simulink model "MIMO_FIXED"  (R2017a)
settings: Solver=VariableStepAuto  StartTime=0.0  StopTime=1000  RelTol=1e-3
libraries: dspsigops x80, commchan3 x4, commdigbbndpm3 x2, commfilt2 x2, commsink2 x1, commutil2 x1
(part 2 of 6)

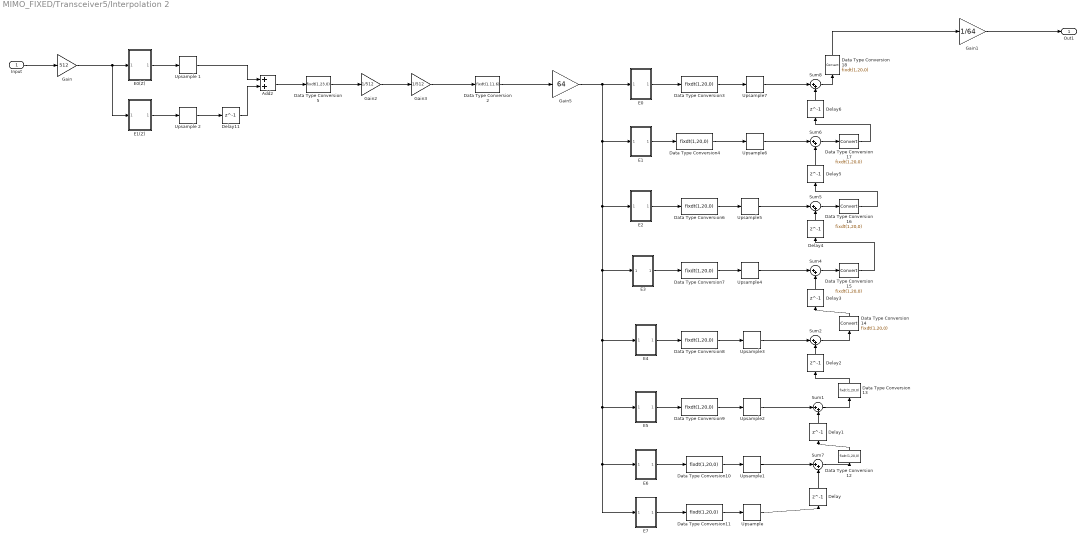
== system MIMO_FIXED/Transceiver5/Interpolation 2 ==
  Input : Inport
  Add2 : Sum
  Data Type Conversion{3..4,6..18} (15 alike) : DataTypeConversion  OutDataTypeStr=fixdt(1,20,0)  SaturateOnIntegerOverflow=on
  Data Type Conversion2 : DataTypeConversion  OutDataTypeStr=fixdt(1,11,6)  SaturateOnIntegerOverflow=on
  Data Type Conversion5 : DataTypeConversion  OutDataTypeStr=fixdt(1,23,0)  SaturateOnIntegerOverflow=on
  Delay{,1..6,11} (8 alike) : Delay  DelayLength=1
  E0 : Subsystem
  E0(Z) : Subsystem
  E1 : Subsystem
  E1(Z) : Subsystem
  E2 : Subsystem
  E3 : Subsystem
  E4 : Subsystem
  E5 : Subsystem
  E6 : Subsystem
  E7 : Subsystem
  Gain : Gain  Gain=512
  Gain1 : Gain  Gain=1/64
  Gain2 : Gain  Gain=1/512
  Gain3 : Gain  Gain=1/512
  Gain5 : Gain  Gain=64
  Sum{1..2,4..8} (7 alike) : Sum  Inputs=|++
  Upsample{,1..7} (8 alike) : dspsigops/Upsample  N=8  phase=0  RateOptions=Allow multirate processing  ic=0  mode=Unused parameter value
  Upsample 1 : dspsigops/Upsample  N=2  phase=0  RateOptions=Allow multirate processing  ic=0  mode=Unused parameter value
  Upsample 2 : dspsigops/Upsample  N=2  phase=0  RateOptions=Allow multirate processing  ic=0  mode=Unused parameter value
  Out1 : Outport
  wires:
  Upsample/1 -> Delay/1
  Delay5/1 -> Sum6/2
  Upsample6/1 -> Sum6/1
  Delay4/1 -> Sum5/2
  Delay3/1 -> Sum4/2
  Sum6/1 -> Data Type Conversion17/1
  Upsample1/1 -> Sum7/1
  Upsample2/1 -> Sum1/1
  Input/1 -> Gain/1
  Upsample 2/1 -> Delay11/1
  Delay6/1 -> Sum8/2
  E0/1(Out1) -> Data Type Conversion3/1
  Delay/1 -> Sum7/2
  E1/1(Out1) -> Data Type Conversion4/1
  Delay1/1 -> Sum1/2
  Sum5/1 -> Data Type Conversion16/1
  Sum4/1 -> Data Type Conversion15/1
  Upsample5/1 -> Sum5/1
  Upsample 1/1 -> Add2/1
  Upsample4/1 -> Sum4/1
  Delay11/1 -> Add2/2
  Sum2/1 -> Data Type Conversion14/1
  E3/1(Out1) -> Data Type Conversion7/1
  Delay2/1 -> Sum2/2
  Upsample7/1 -> Sum8/1
  Upsample3/1 -> Sum2/1
  E2/1(Out1) -> Data Type Conversion6/1
  E4/1(Out1) -> Data Type Conversion8/1
  E0(Z)/1(Out1) -> Upsample 1/1
  Data Type Conversion3/1 -> Upsample7/1
  Data Type Conversion4/1 -> Upsample6/1
  Data Type Conversion6/1 -> Upsample5/1
  Data Type Conversion7/1 -> Upsample4/1
  Data Type Conversion8/1 -> Upsample3/1
  Data Type Conversion9/1 -> Upsample2/1
  Data Type Conversion10/1 -> Upsample1/1
  Data Type Conversion11/1 -> Upsample/1
  Data Type Conversion12/1 -> Delay1/1
  Sum7/1 -> Data Type Conversion12/1
  Data Type Conversion13/1 -> Delay2/1
  Data Type Conversion14/1 -> Delay3/1
  Sum1/1 -> Data Type Conversion13/1
  Data Type Conversion15/1 -> Delay4/1
  Data Type Conversion16/1 -> Delay5/1
  Data Type Conversion17/1 -> Delay6/1
  Data Type Conversion18/1 -> Gain1/1
  Sum8/1 -> Data Type Conversion18/1
  E5/1(Out1) -> Data Type Conversion9/1
  E6/1(Out1) -> Data Type Conversion10/1
  E7/1(Out1) -> Data Type Conversion11/1
  Gain5/1 -> E0/1(In1), E7/1(In1), E6/1(In1), E5/1(In1), E4/1(In1), E3/1(In1), E2/1(In1), E1/1(In1)
  Gain1/1 -> Out1/1
  Gain/1 -> E0(Z)/1(Input), E1(Z)/1(Input1)
  Data Type Conversion2/1 -> Gain5/1
  Gain2/1 -> Gain3/1
  E1(Z)/1(Output) -> Upsample 2/1
  Gain3/1 -> Data Type Conversion2/1
  Add2/1 -> Data Type Conversion5/1
  Data Type Conversion5/1 -> Gain2/1

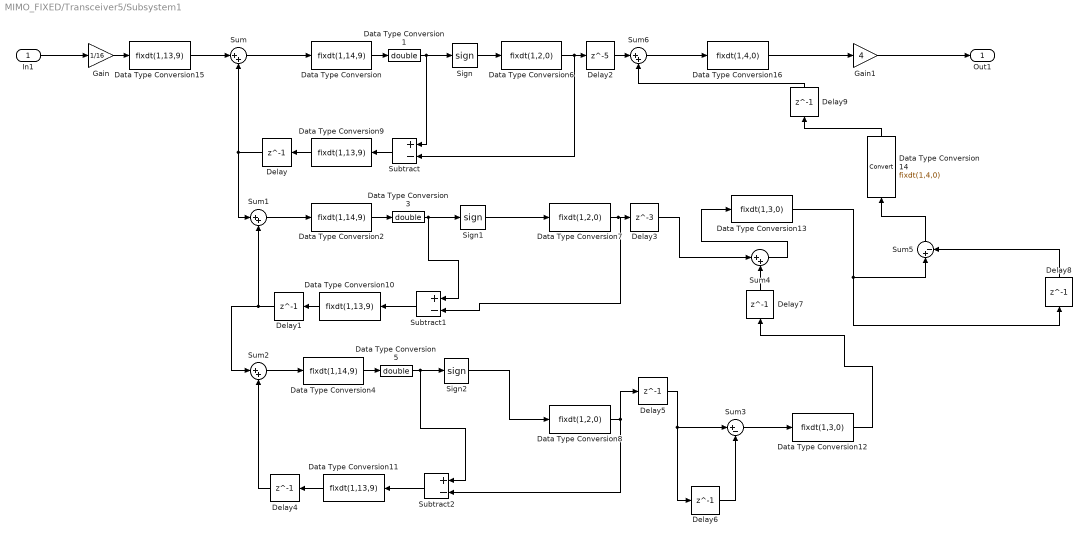
== system MIMO_FIXED/Transceiver5/Subsystem1 ==
  In1 : Inport
  Data Type Conversion : DataTypeConversion  OutDataTypeStr=fixdt(1,14,9)
  Data Type Conversion1 : DataTypeConversion  OutDataTypeStr=double
  Data Type Conversion{9..11,15} (4 alike) : DataTypeConversion  OutDataTypeStr=fixdt(1,13,9)
  Data Type Conversion12 : DataTypeConversion  OutDataTypeStr=fixdt(1,3,0)
  Data Type Conversion13 : DataTypeConversion  OutDataTypeStr=fixdt(1,3,0)
  Data Type Conversion14 : DataTypeConversion  OutDataTypeStr=fixdt(1,4,0)
  Data Type Conversion16 : DataTypeConversion  OutDataTypeStr=fixdt(1,4,0)
  Data Type Conversion2 : DataTypeConversion  OutDataTypeStr=fixdt(1,14,9)
  Data Type Conversion3 : DataTypeConversion  OutDataTypeStr=double
  Data Type Conversion4 : DataTypeConversion  OutDataTypeStr=fixdt(1,14,9)
  Data Type Conversion5 : DataTypeConversion  OutDataTypeStr=double
  Data Type Conversion6 : DataTypeConversion  OutDataTypeStr=fixdt(1,2,0)
  Data Type Conversion7 : DataTypeConversion  OutDataTypeStr=fixdt(1,2,0)
  Data Type Conversion8 : DataTypeConversion  OutDataTypeStr=fixdt(1,2,0)
  Delay{,1,4..9} (8 alike) : Delay  DelayLength=1
  Delay2 : Delay  DelayLength=5
  Delay3 : Delay  DelayLength=3
  Gain : Gain  Gain=1/16
  Gain1 : Gain  Gain=4
  Sign : Signum
  Sign1 : Signum
  Sign2 : Signum
  Subtract : Sum  Inputs=+-
  Subtract1 : Sum  Inputs=+-
  Subtract2 : Sum  Inputs=+-
  Sum{,1..2,4,6} (5 alike) : Sum  Inputs=|++
  Sum3 : Sum  Inputs=|+-
  Sum5 : Sum  Inputs=|+-
  Out1 : Outport
  wires:
  Sum/1 -> Data Type Conversion/1
  Sum2/1 -> Data Type Conversion4/1
  Delay4/1 -> Sum2/2
  Delay8/1 -> Sum5/2
  Sum4/1 -> Data Type Conversion13/1
  Subtract/1 -> Data Type Conversion9/1
  Delay5/1 -> Sum3/1, Delay6/1
  Sign1/1 -> Data Type Conversion7/1
  Delay1/1 -> Sum1/2, Sum2/1
  Sum1/1 -> Data Type Conversion2/1
  Subtract1/1 -> Data Type Conversion10/1
  Sum3/1 -> Data Type Conversion12/1
  Delay/1 -> Sum/2, Sum1/1
  Delay3/1 -> Sum4/1
  Delay7/1 -> Sum4/2
  Subtract2/1 -> Data Type Conversion11/1
  Delay6/1 -> Sum3/2
  Sum5/1 -> Data Type Conversion14/1
  Delay2/1 -> Sum6/1
  Delay9/1 -> Sum6/2
  In1/1 -> Gain/1
  Sum6/1 -> Data Type Conversion16/1
  Data Type Conversion/1 -> Data Type Conversion1/1
  Data Type Conversion1/1 -> Subtract/1, Sign/1
  Data Type Conversion2/1 -> Data Type Conversion3/1
  Data Type Conversion4/1 -> Data Type Conversion5/1
  Data Type Conversion6/1 -> Subtract/2, Delay2/1
  Data Type Conversion7/1 -> Subtract1/2, Delay3/1
  Data Type Conversion8/1 -> Delay5/1, Subtract2/2
  Data Type Conversion9/1 -> Delay/1
  Data Type Conversion10/1 -> Delay1/1
  Data Type Conversion11/1 -> Delay4/1
  Data Type Conversion12/1 -> Delay7/1
  Data Type Conversion13/1 -> Sum5/1, Delay8/1
  Data Type Conversion14/1 -> Delay9/1
  Gain/1 -> Data Type Conversion15/1
  Gain1/1 -> Out1/1
  Data Type Conversion15/1 -> Sum/1
  Data Type Conversion16/1 -> Gain1/1
  Sign/1 -> Data Type Conversion6/1
  Data Type Conversion3/1 -> Sign1/1, Subtract1/1
  Data Type Conversion5/1 -> Sign2/1, Subtract2/1
  Sign2/1 -> Data Type Conversion8/1

== system MIMO_FIXED/Transceiver5/Subsystem2 ==
  In1 : Inport
  Data Type Conversion : DataTypeConversion  OutDataTypeStr=fixdt(1,14,9)
  Data Type Conversion1 : DataTypeConversion  OutDataTypeStr=double
  Data Type Conversion{9..11,15} (4 alike) : DataTypeConversion  OutDataTypeStr=fixdt(1,13,9)
  Data Type Conversion12 : DataTypeConversion  OutDataTypeStr=fixdt(1,3,0)
  Data Type Conversion13 : DataTypeConversion  OutDataTypeStr=fixdt(1,3,0)
  Data Type Conversion14 : DataTypeConversion  OutDataTypeStr=fixdt(1,4,0)
  Data Type Conversion16 : DataTypeConversion  OutDataTypeStr=fixdt(1,4,0)
  Data Type Conversion2 : DataTypeConversion  OutDataTypeStr=fixdt(1,14,9)
  Data Type Conversion3 : DataTypeConversion  OutDataTypeStr=double
  Data Type Conversion4 : DataTypeConversion  OutDataTypeStr=fixdt(1,14,9)
  Data Type Conversion5 : DataTypeConversion  OutDataTypeStr=double
  Data Type Conversion6 : DataTypeConversion  OutDataTypeStr=fixdt(1,2,0)
  Data Type Conversion7 : DataTypeConversion  OutDataTypeStr=fixdt(1,2,0)
  Data Type Conversion8 : DataTypeConversion  OutDataTypeStr=fixdt(1,2,0)
  Delay{,1,4..9} (8 alike) : Delay  DelayLength=1
  Delay2 : Delay  DelayLength=5
  Delay3 : Delay  DelayLength=3
  Gain : Gain  Gain=1/16
  Gain1 : Gain  Gain=4
  Sign : Signum
  Sign1 : Signum
  Sign2 : Signum
  Subtract : Sum  Inputs=+-
  Subtract1 : Sum  Inputs=+-
  Subtract2 : Sum  Inputs=+-
  Sum{,1..2,4,6} (5 alike) : Sum  Inputs=|++
  Sum3 : Sum  Inputs=|+-
  Sum5 : Sum  Inputs=|+-
  Out1 : Outport
  wires:
  Sum/1 -> Data Type Conversion/1
  Sum2/1 -> Data Type Conversion4/1
  Delay4/1 -> Sum2/2
  Delay8/1 -> Sum5/2
  Sum4/1 -> Data Type Conversion13/1
  Subtract/1 -> Data Type Conversion9/1
  Delay5/1 -> Sum3/1, Delay6/1
  Sign1/1 -> Data Type Conversion7/1
  Delay1/1 -> Sum1/2, Sum2/1
  Sum1/1 -> Data Type Conversion2/1
  Subtract1/1 -> Data Type Conversion10/1
  Sum3/1 -> Data Type Conversion12/1
  Delay/1 -> Sum/2, Sum1/1
  Delay3/1 -> Sum4/1
  Delay7/1 -> Sum4/2
  Subtract2/1 -> Data Type Conversion11/1
  Delay6/1 -> Sum3/2
  Sum5/1 -> Data Type Conversion14/1
  Delay2/1 -> Sum6/1
  Delay9/1 -> Sum6/2
  In1/1 -> Gain/1
  Sum6/1 -> Data Type Conversion16/1
  Data Type Conversion/1 -> Data Type Conversion1/1
  Data Type Conversion1/1 -> Subtract/1, Sign/1
  Data Type Conversion2/1 -> Data Type Conversion3/1
  Data Type Conversion4/1 -> Data Type Conversion5/1
  Data Type Conversion6/1 -> Subtract/2, Delay2/1
  Data Type Conversion7/1 -> Subtract1/2, Delay3/1
  Data Type Conversion8/1 -> Delay5/1, Subtract2/2
  Data Type Conversion9/1 -> Delay/1
  Data Type Conversion10/1 -> Delay1/1
  Data Type Conversion11/1 -> Delay4/1
  Data Type Conversion12/1 -> Delay7/1
  Data Type Conversion13/1 -> Sum5/1, Delay8/1
  Data Type Conversion14/1 -> Delay9/1
  Gain/1 -> Data Type Conversion15/1
  Gain1/1 -> Out1/1
  Data Type Conversion15/1 -> Sum/1
  Data Type Conversion16/1 -> Gain1/1
  Sign/1 -> Data Type Conversion6/1
  Data Type Conversion3/1 -> Sign1/1, Subtract1/1
  Data Type Conversion5/1 -> Sign2/1, Subtract2/1
  Sign2/1 -> Data Type Conversion8/1

== system MIMO_FIXED/Transceiver6/ADC 1 ==
  In1 : Inport
  SigmaDelta ADC : Subsystem
  Switch : Switch  Criteria=u2 > Threshold  OutDataTypeStr=boolean
  Zero : Constant  Value=0
  bits 1&0 : Outport
  wires:
  SigmaDelta ADC/1(Out) -> Switch/1, Switch/2
  Zero/1 -> Switch/3
  In1/1 -> SigmaDelta ADC/1(In)
  Switch/1 -> bits 1&0/1

== system MIMO_FIXED/Transceiver6/CWM_RX2 ==
  In1 : Inport
  I_DDC : Inport  Port=2
  Q_DDC : Inport  Port=3
  Add : Sum
  Add1 : Sum  Inputs=-+
  Data Type Conversion{,1..9} (10 alike) : DataTypeConversion  OutDataTypeStr=fixdt(1,6,4)  SaturateOnIntegerOverflow=on
  Gain{,2,4,6} (4 alike) : Gain  Gain=-1
  Gain{1,3,5,7} (4 alike) : Gain
  Multiport Switch{,1,4..5} (4 alike) : MultiPortSwitch  DataPortOrder=Zero-based contiguous  Inputs=2  zeroidx=on  RndMeth=Nearest
  Trigonometric Function{,1,4..5} (4 alike) : Trigonometry
  Trigonometric Function{2..3,6..7} (4 alike) : Trigonometry  Operator=cos
  I` : Outport
  Q` : Outport  Port=2
  wires:
  Multiport Switch/1 -> Add1/1
  Add/1 -> Data Type Conversion8/1
  I_DDC/1 -> Multiport Switch1/1, Multiport Switch/1
  Gain2/1 -> Data Type Conversion6/1
  Trigonometric Function5/1 -> Gain5/1
  Data Type Conversion6/1 -> Multiport Switch1/2
  Data Type Conversion7/1 -> Multiport Switch/3
  Gain5/1 -> Data Type Conversion3/1
  Gain4/1 -> Data Type Conversion4/1
  Trigonometric Function1/1 -> Gain1/1
  Data Type Conversion2/1 -> Multiport Switch5/2
  Gain1/1 -> Data Type Conversion7/1
  Gain3/1 -> Data Type Conversion5/1
  Trigonometric Function3/1 -> Gain3/1
  Add1/1 -> Data Type Conversion9/1
  Gain/1 -> Data Type Conversion/1
  Trigonometric Function2/1 -> Gain2/1
  In1/1 -> Trigonometric Function3/1, Trigonometric Function6/1, Trigonometric Function7/1, Trigonometric Function5/1, Trigonometric Function4/1, Trigonometric Function2/1, Trigonometric Function1/1, Trigonometric Function/1
  Q_DDC/1 -> Multiport Switch5/1, Multiport Switch4/1
  Data Type Conversion1/1 -> Multiport Switch5/3
  Data Type Conversion4/1 -> Multiport Switch4/2
  Trigonometric Function6/1 -> Gain6/1
  Gain7/1 -> Data Type Conversion1/1
  Trigonometric Function4/1 -> Gain4/1
  Trigonometric Function/1 -> Gain/1
  Multiport Switch1/1 -> Add/1
  Multiport Switch4/1 -> Add/2
  Trigonometric Function7/1 -> Gain7/1
  Multiport Switch5/1 -> Add1/2
  Data Type Conversion3/1 -> Multiport Switch4/3
  Gain6/1 -> Data Type Conversion2/1
  Data Type Conversion/1 -> Multiport Switch/2
  Data Type Conversion5/1 -> Multiport Switch1/3
  Data Type Conversion8/1 -> I`/1
  Data Type Conversion9/1 -> Q`/1

== system MIMO_FIXED/Transceiver6/CWM_TX_Chain_1 ==
  PHI : Inport
  Processor_I : Inport  Port=2
  Processor_Q : Inport  Port=3
  Add : Sum  OutDataTypeStr=double  RndMeth=Round  SaturateOnIntegerOverflow=on
  Add1 : Sum  OutDataTypeStr=double
  Data Type Conversion : DataTypeConversion  OutDataTypeStr=fixdt(1,6,4)  SaturateOnIntegerOverflow=on
  Data Type Conversion1 : DataTypeConversion  OutDataTypeStr=fixdt(1,6,4)  RndMeth=Round  SaturateOnIntegerOverflow=on
  Data Type Conversion12 : DataTypeConversion  OutDataTypeStr=fixdt(1,16,9)  SaturateOnIntegerOverflow=on
  Data Type Conversion2 : DataTypeConversion  OutDataTypeStr=fixdt(1,6,4)  RndMeth=Round  SaturateOnIntegerOverflow=on
  Data Type Conversion3 : DataTypeConversion  OutDataTypeStr=fixdt(1,6,4)  SaturateOnIntegerOverflow=on
  Data Type Conversion4 : DataTypeConversion  OutDataTypeStr=fixdt(1,16,7)  SaturateOnIntegerOverflow=on
  Data Type Conversion5 : DataTypeConversion  OutDataTypeStr=fixdt(1,16,9)  SaturateOnIntegerOverflow=on
  Data Type Conversion6 : DataTypeConversion  OutDataTypeStr=fixdt(1,16,9)  SaturateOnIntegerOverflow=on
  Data Type Conversion7 : DataTypeConversion  OutDataTypeStr=fixdt(1,18,9)  SaturateOnIntegerOverflow=on
  Data Type Conversion8 : DataTypeConversion  OutDataTypeStr=fixdt(1,18,9)  SaturateOnIntegerOverflow=on
  Gain1 : Gain  Gain=-1
  Gain2 : Gain
  Gain3 : Gain
  Gain4 : Gain
  Product{,1..3} (4 alike) : Product
  Trigonometric Function1 : Trigonometry
  Trigonometric Function2 : Trigonometry  Operator=cos
  Trigonometric Function3 : Trigonometry  Operator=cos
  Trigonometric Function4 : Trigonometry
  I_1 : Outport
  Q_1 : Outport  Port=2
  wires:
  Trigonometric Function2/1 -> Gain2/1
  Gain2/1 -> Data Type Conversion/1
  Processor_Q/1 -> Product1/2, Product3/2
  Processor_I/1 -> Product2/1, Product/1
  Gain1/1 -> Data Type Conversion1/1
  Product/1 -> Data Type Conversion12/1
  Trigonometric Function1/1 -> Gain1/1
  PHI/1 -> Trigonometric Function2/1, Trigonometric Function1/1, Trigonometric Function4/1, Trigonometric Function3/1
  Data Type Conversion1/1 -> Product1/1
  Gain3/1 -> Data Type Conversion3/1
  Product2/1 -> Data Type Conversion5/1
  Data Type Conversion/1 -> Product/2
  Data Type Conversion2/1 -> Product2/2
  Data Type Conversion3/1 -> Product3/1
  Product3/1 -> Data Type Conversion6/1
  Trigonometric Function3/1 -> Gain3/1
  Product1/1 -> Data Type Conversion4/1
  Gain4/1 -> Data Type Conversion2/1
  Trigonometric Function4/1 -> Gain4/1
  Add1/1 -> Data Type Conversion8/1
  Data Type Conversion7/1 -> I_1/1
  Data Type Conversion8/1 -> Q_1/1
  Data Type Conversion12/1 -> Add/1
  Data Type Conversion4/1 -> Add/2
  Data Type Conversion5/1 -> Add1/1
  Data Type Conversion6/1 -> Add1/2
  Add/1 -> Data Type Conversion7/1

== system MIMO_FIXED/Transceiver6/DDC2 ==
  ODD_I : Inport
  EVEN_Q : Inport  Port=2
  Local_Oscilator1 : DiscretePulseGenerator  PhaseDelay=1  SampleTime=0.02
  Logical Operator : Logic  Operator=NXOR  AllPortsSameDT=off  OutDataTypeStr=boolean
  Logical Operator1 : Logic  Operator=NXOR  AllPortsSameDT=off  OutDataTypeStr=boolean
  NOT : Logic  Operator=NOT  IconShape=distinctive  AllPortsSameDT=off  OutDataTypeStr=boolean
  I_DDC : Outport
  Q_DDC : Outport  Port=2
  wires:
  Logical Operator/1 -> I_DDC/1
  EVEN_Q/1 -> Logical Operator1/2
  ODD_I/1 -> Logical Operator/1
  Logical Operator1/1 -> Q_DDC/1
  Local_Oscilator1/1 -> NOT/1
  NOT/1 -> Logical Operator1/1, Logical Operator/2

== system MIMO_FIXED/Transceiver6/DUC2 ==
  I_1 : Inport
  Q_1 : Inport  Port=2
  -cos : Sin  SineType=Sample based  Frequency=2*pi*100  Phase=pi/2  Samples=4  SampleTime=0.01  Offset=3
  -sin1 : Sin  SineType=Sample based  Frequency=(2*pi*100)/4  Samples=4  SampleTime=.01  Offset=2
  Add : Sum
  Constant : Constant  Value=0
  Constant1 : Constant  Value=0
  Data Type Conversion : DataTypeConversion  OutDataTypeStr=fixdt(1,2,0)  RndMeth=Round
  Data Type Conversion1 : DataTypeConversion  OutDataTypeStr=fixdt(1,2,0)  RndMeth=Round
  Data Type Conversion{2..3,5..6} (4 alike) : DataTypeConversion  OutDataTypeStr=fixdt(1,6,0)
  Data Type Conversion4 : DataTypeConversion  OutDataTypeStr=fixdt(1,7,0)
  Gain : Gain  Gain=-1
  Gain1 : Gain  Gain=-1
  Multiport Switch : MultiPortSwitch  DataPortOrder=Specify indices  DataPortIndices={1,0,-1}  RndMeth=Nearest
  Multiport Switch1 : MultiPortSwitch  DataPortOrder=Specify indices  DataPortIndices={1,0,-1}  RndMeth=Nearest
  Out2 : Outport
  wires:
  Constant/1 -> Multiport Switch1/3
  Q_1/1 -> Multiport Switch/2, Gain1/1
  I_1/1 -> Multiport Switch1/2, Gain/1
  Gain1/1 -> Data Type Conversion2/1
  -sin1/1 -> Data Type Conversion1/1
  -cos/1 -> Data Type Conversion/1
  Multiport Switch/1 -> Data Type Conversion5/1
  Add/1 -> Data Type Conversion4/1
  Multiport Switch1/1 -> Data Type Conversion6/1
  Constant1/1 -> Multiport Switch/3
  Gain/1 -> Data Type Conversion3/1
  Data Type Conversion/1 -> Multiport Switch1/1
  Data Type Conversion1/1 -> Multiport Switch/1
  Data Type Conversion2/1 -> Multiport Switch/4
  Data Type Conversion3/1 -> Multiport Switch1/4
  Data Type Conversion6/1 -> Add/1
  Data Type Conversion5/1 -> Add/2
  Data Type Conversion4/1 -> Out2/1

== system MIMO_FIXED/Transceiver6/Inter_Lever2 ==
  bits 1&0 : Inport
  Delay1 : Delay  DelayLength=1  InitialCondition=0
  Delay2 : Delay  DelayLength=1  InitialCondition=0
  Downsample : DownSample  RateOptions=Allow multirate processing
  Downsample1 : DownSample  RateOptions=Allow multirate processing
  ODD_I : Outport
  EVEN_Q : Outport  Port=2
  wires:
  Delay1/1 -> Downsample1/1
  Downsample/1 -> Delay2/1
  Downsample1/1 -> EVEN_Q/1
  bits 1&0/1 -> Delay1/1, Downsample/1
  Delay2/1 -> ODD_I/1

== system MIMO_FIXED/Transceiver6/Interpolation 1 ==
  Input : Inport
  Data Type Conversion2 : DataTypeConversion  OutDataTypeStr=fixdt(1,11,6)  SaturateOnIntegerOverflow=on
  Data Type Conversion5 : DataTypeConversion  OutDataTypeStr=fixdt(1,23,0)  SaturateOnIntegerOverflow=on
  Gain : Gain  Gain=512
  Gain1 : Gain  Gain=1/64
  Gain2 : Gain  Gain=1/512
  Gain3 : Gain  Gain=1/512
  Gain5 : Gain  Gain=64
  Half_band : Subsystem
  comb_filter : Subsystem
  Out1 : Outport
  wires:
  Input/1 -> Gain/1
  Gain5/1 -> comb_filter/1(In1)
  Gain1/1 -> Out1/1
  Data Type Conversion2/1 -> Gain5/1
  Gain2/1 -> Gain3/1
  Gain3/1 -> Data Type Conversion2/1
  Data Type Conversion5/1 -> Gain2/1
  Gain/1 -> Half_band/1(Input)
  Half_band/1(Out1) -> Data Type Conversion5/1
  comb_filter/1(Out1) -> Gain1/1

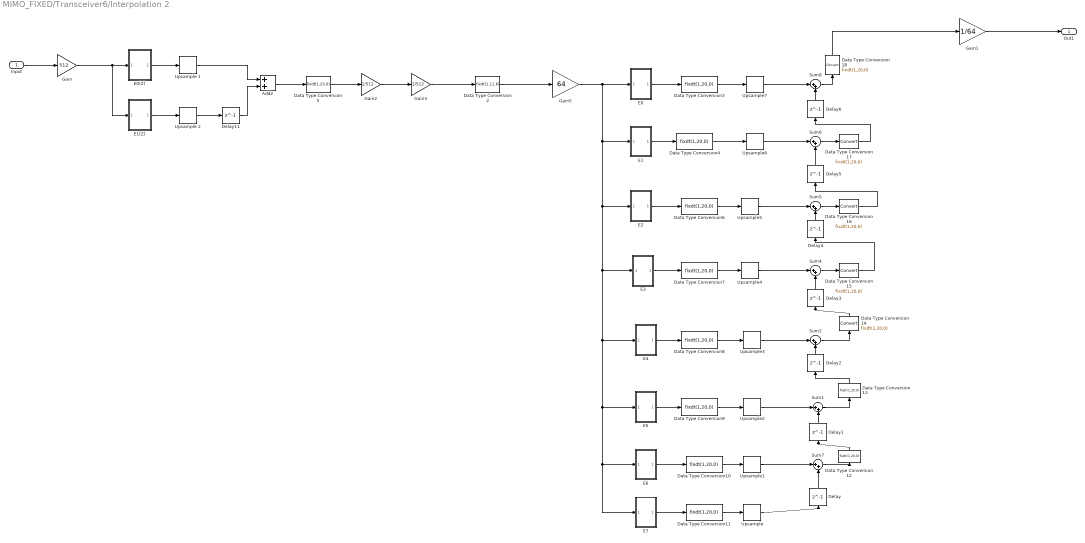
== system MIMO_FIXED/Transceiver6/Interpolation 2 ==
  Input : Inport
  Add2 : Sum
  Data Type Conversion{3..4,6..18} (15 alike) : DataTypeConversion  OutDataTypeStr=fixdt(1,20,0)  SaturateOnIntegerOverflow=on
  Data Type Conversion2 : DataTypeConversion  OutDataTypeStr=fixdt(1,11,6)  SaturateOnIntegerOverflow=on
  Data Type Conversion5 : DataTypeConversion  OutDataTypeStr=fixdt(1,23,0)  SaturateOnIntegerOverflow=on
  Delay{,1..6,11} (8 alike) : Delay  DelayLength=1
  E0 : Subsystem
  E0(Z) : Subsystem
  E1 : Subsystem
  E1(Z) : Subsystem
  E2 : Subsystem
  E3 : Subsystem
  E4 : Subsystem
  E5 : Subsystem
  E6 : Subsystem
  E7 : Subsystem
  Gain : Gain  Gain=512
  Gain1 : Gain  Gain=1/64
  Gain2 : Gain  Gain=1/512
  Gain3 : Gain  Gain=1/512
  Gain5 : Gain  Gain=64
  Sum{1..2,4..8} (7 alike) : Sum  Inputs=|++
  Upsample{,1..7} (8 alike) : dspsigops/Upsample  N=8  phase=0  RateOptions=Allow multirate processing  ic=0  mode=Unused parameter value
  Upsample 1 : dspsigops/Upsample  N=2  phase=0  RateOptions=Allow multirate processing  ic=0  mode=Unused parameter value
  Upsample 2 : dspsigops/Upsample  N=2  phase=0  RateOptions=Allow multirate processing  ic=0  mode=Unused parameter value
  Out1 : Outport
  wires:
  Upsample/1 -> Delay/1
  Delay5/1 -> Sum6/2
  Upsample6/1 -> Sum6/1
  Delay4/1 -> Sum5/2
  Delay3/1 -> Sum4/2
  Sum6/1 -> Data Type Conversion17/1
  Upsample1/1 -> Sum7/1
  Upsample2/1 -> Sum1/1
  Input/1 -> Gain/1
  Upsample 2/1 -> Delay11/1
  Delay6/1 -> Sum8/2
  E0/1(Out1) -> Data Type Conversion3/1
  Delay/1 -> Sum7/2
  E1/1(Out1) -> Data Type Conversion4/1
  Delay1/1 -> Sum1/2
  Sum5/1 -> Data Type Conversion16/1
  Sum4/1 -> Data Type Conversion15/1
  Upsample5/1 -> Sum5/1
  Upsample 1/1 -> Add2/1
  Upsample4/1 -> Sum4/1
  Delay11/1 -> Add2/2
  Sum2/1 -> Data Type Conversion14/1
  E3/1(Out1) -> Data Type Conversion7/1
  Delay2/1 -> Sum2/2
  Upsample7/1 -> Sum8/1
  Upsample3/1 -> Sum2/1
  E2/1(Out1) -> Data Type Conversion6/1
  E4/1(Out1) -> Data Type Conversion8/1
  E0(Z)/1(Out1) -> Upsample 1/1
  Data Type Conversion3/1 -> Upsample7/1
  Data Type Conversion4/1 -> Upsample6/1
  Data Type Conversion6/1 -> Upsample5/1
  Data Type Conversion7/1 -> Upsample4/1
  Data Type Conversion8/1 -> Upsample3/1
  Data Type Conversion9/1 -> Upsample2/1
  Data Type Conversion10/1 -> Upsample1/1
  Data Type Conversion11/1 -> Upsample/1
  Data Type Conversion12/1 -> Delay1/1
  Sum7/1 -> Data Type Conversion12/1
  Data Type Conversion13/1 -> Delay2/1
  Data Type Conversion14/1 -> Delay3/1
  Sum1/1 -> Data Type Conversion13/1
  Data Type Conversion15/1 -> Delay4/1
  Data Type Conversion16/1 -> Delay5/1
  Data Type Conversion17/1 -> Delay6/1
  Data Type Conversion18/1 -> Gain1/1
  Sum8/1 -> Data Type Conversion18/1
  E5/1(Out1) -> Data Type Conversion9/1
  E6/1(Out1) -> Data Type Conversion10/1
  E7/1(Out1) -> Data Type Conversion11/1
  Gain5/1 -> E0/1(In1), E7/1(In1), E6/1(In1), E5/1(In1), E4/1(In1), E3/1(In1), E2/1(In1), E1/1(In1)
  Gain1/1 -> Out1/1
  Gain/1 -> E0(Z)/1(Input), E1(Z)/1(Input1)
  Data Type Conversion2/1 -> Gain5/1
  Gain2/1 -> Gain3/1
  E1(Z)/1(Output) -> Upsample 2/1
  Gain3/1 -> Data Type Conversion2/1
  Add2/1 -> Data Type Conversion5/1
  Data Type Conversion5/1 -> Gain2/1

== system MIMO_FIXED/Transceiver6/Subsystem1 ==
  In1 : Inport
  Data Type Conversion : DataTypeConversion  OutDataTypeStr=fixdt(1,14,9)
  Data Type Conversion1 : DataTypeConversion  OutDataTypeStr=double
  Data Type Conversion{9..11,15} (4 alike) : DataTypeConversion  OutDataTypeStr=fixdt(1,13,9)
  Data Type Conversion12 : DataTypeConversion  OutDataTypeStr=fixdt(1,3,0)
  Data Type Conversion13 : DataTypeConversion  OutDataTypeStr=fixdt(1,3,0)
  Data Type Conversion14 : DataTypeConversion  OutDataTypeStr=fixdt(1,4,0)
  Data Type Conversion16 : DataTypeConversion  OutDataTypeStr=fixdt(1,4,0)
  Data Type Conversion2 : DataTypeConversion  OutDataTypeStr=fixdt(1,14,9)
  Data Type Conversion3 : DataTypeConversion  OutDataTypeStr=double
  Data Type Conversion4 : DataTypeConversion  OutDataTypeStr=fixdt(1,14,9)
  Data Type Conversion5 : DataTypeConversion  OutDataTypeStr=double
  Data Type Conversion6 : DataTypeConversion  OutDataTypeStr=fixdt(1,2,0)
  Data Type Conversion7 : DataTypeConversion  OutDataTypeStr=fixdt(1,2,0)
  Data Type Conversion8 : DataTypeConversion  OutDataTypeStr=fixdt(1,2,0)
  Delay{,1,4..9} (8 alike) : Delay  DelayLength=1
  Delay2 : Delay  DelayLength=5
  Delay3 : Delay  DelayLength=3
  Gain : Gain  Gain=1/16
  Gain1 : Gain  Gain=4
  Sign : Signum
  Sign1 : Signum
  Sign2 : Signum
  Subtract : Sum  Inputs=+-
  Subtract1 : Sum  Inputs=+-
  Subtract2 : Sum  Inputs=+-
  Sum{,1..2,4,6} (5 alike) : Sum  Inputs=|++
  Sum3 : Sum  Inputs=|+-
  Sum5 : Sum  Inputs=|+-
  Out1 : Outport
  wires:
  Sum/1 -> Data Type Conversion/1
  Sum2/1 -> Data Type Conversion4/1
  Delay4/1 -> Sum2/2
  Delay8/1 -> Sum5/2
  Sum4/1 -> Data Type Conversion13/1
  Subtract/1 -> Data Type Conversion9/1
  Delay5/1 -> Sum3/1, Delay6/1
  Sign1/1 -> Data Type Conversion7/1
  Delay1/1 -> Sum1/2, Sum2/1
  Sum1/1 -> Data Type Conversion2/1
  Subtract1/1 -> Data Type Conversion10/1
  Sum3/1 -> Data Type Conversion12/1
  Delay/1 -> Sum/2, Sum1/1
  Delay3/1 -> Sum4/1
  Delay7/1 -> Sum4/2
  Subtract2/1 -> Data Type Conversion11/1
  Delay6/1 -> Sum3/2
  Sum5/1 -> Data Type Conversion14/1
  Delay2/1 -> Sum6/1
  Delay9/1 -> Sum6/2
  In1/1 -> Gain/1
  Sum6/1 -> Data Type Conversion16/1
  Data Type Conversion/1 -> Data Type Conversion1/1
  Data Type Conversion1/1 -> Subtract/1, Sign/1
  Data Type Conversion2/1 -> Data Type Conversion3/1
  Data Type Conversion4/1 -> Data Type Conversion5/1
  Data Type Conversion6/1 -> Subtract/2, Delay2/1
  Data Type Conversion7/1 -> Subtract1/2, Delay3/1
  Data Type Conversion8/1 -> Delay5/1, Subtract2/2
  Data Type Conversion9/1 -> Delay/1
  Data Type Conversion10/1 -> Delay1/1
  Data Type Conversion11/1 -> Delay4/1
  Data Type Conversion12/1 -> Delay7/1
  Data Type Conversion13/1 -> Sum5/1, Delay8/1
  Data Type Conversion14/1 -> Delay9/1
  Gain/1 -> Data Type Conversion15/1
  Gain1/1 -> Out1/1
  Data Type Conversion15/1 -> Sum/1
  Data Type Conversion16/1 -> Gain1/1
  Sign/1 -> Data Type Conversion6/1
  Data Type Conversion3/1 -> Sign1/1, Subtract1/1
  Data Type Conversion5/1 -> Sign2/1, Subtract2/1
  Sign2/1 -> Data Type Conversion8/1

== system MIMO_FIXED/Transceiver6/Subsystem2 ==
  In1 : Inport
  Data Type Conversion : DataTypeConversion  OutDataTypeStr=fixdt(1,14,9)
  Data Type Conversion1 : DataTypeConversion  OutDataTypeStr=double
  Data Type Conversion{9..11,15} (4 alike) : DataTypeConversion  OutDataTypeStr=fixdt(1,13,9)
  Data Type Conversion12 : DataTypeConversion  OutDataTypeStr=fixdt(1,3,0)
  Data Type Conversion13 : DataTypeConversion  OutDataTypeStr=fixdt(1,3,0)
  Data Type Conversion14 : DataTypeConversion  OutDataTypeStr=fixdt(1,4,0)
  Data Type Conversion16 : DataTypeConversion  OutDataTypeStr=fixdt(1,4,0)
  Data Type Conversion2 : DataTypeConversion  OutDataTypeStr=fixdt(1,14,9)
  Data Type Conversion3 : DataTypeConversion  OutDataTypeStr=double
  Data Type Conversion4 : DataTypeConversion  OutDataTypeStr=fixdt(1,14,9)
  Data Type Conversion5 : DataTypeConversion  OutDataTypeStr=double
  Data Type Conversion6 : DataTypeConversion  OutDataTypeStr=fixdt(1,2,0)
  Data Type Conversion7 : DataTypeConversion  OutDataTypeStr=fixdt(1,2,0)
  Data Type Conversion8 : DataTypeConversion  OutDataTypeStr=fixdt(1,2,0)
  Delay{,1,4..9} (8 alike) : Delay  DelayLength=1
  Delay2 : Delay  DelayLength=5
  Delay3 : Delay  DelayLength=3
  Gain : Gain  Gain=1/16
  Gain1 : Gain  Gain=4
  Sign : Signum
  Sign1 : Signum
  Sign2 : Signum
  Subtract : Sum  Inputs=+-
  Subtract1 : Sum  Inputs=+-
  Subtract2 : Sum  Inputs=+-
  Sum{,1..2,4,6} (5 alike) : Sum  Inputs=|++
  Sum3 : Sum  Inputs=|+-
  Sum5 : Sum  Inputs=|+-
  Out1 : Outport
  wires:
  Sum/1 -> Data Type Conversion/1
  Sum2/1 -> Data Type Conversion4/1
  Delay4/1 -> Sum2/2
  Delay8/1 -> Sum5/2
  Sum4/1 -> Data Type Conversion13/1
  Subtract/1 -> Data Type Conversion9/1
  Delay5/1 -> Sum3/1, Delay6/1
  Sign1/1 -> Data Type Conversion7/1
  Delay1/1 -> Sum1/2, Sum2/1
  Sum1/1 -> Data Type Conversion2/1
  Subtract1/1 -> Data Type Conversion10/1
  Sum3/1 -> Data Type Conversion12/1
  Delay/1 -> Sum/2, Sum1/1
  Delay3/1 -> Sum4/1
  Delay7/1 -> Sum4/2
  Subtract2/1 -> Data Type Conversion11/1
  Delay6/1 -> Sum3/2
  Sum5/1 -> Data Type Conversion14/1
  Delay2/1 -> Sum6/1
  Delay9/1 -> Sum6/2
  In1/1 -> Gain/1
  Sum6/1 -> Data Type Conversion16/1
  Data Type Conversion/1 -> Data Type Conversion1/1
  Data Type Conversion1/1 -> Subtract/1, Sign/1
  Data Type Conversion2/1 -> Data Type Conversion3/1
  Data Type Conversion4/1 -> Data Type Conversion5/1
  Data Type Conversion6/1 -> Subtract/2, Delay2/1
  Data Type Conversion7/1 -> Subtract1/2, Delay3/1
  Data Type Conversion8/1 -> Delay5/1, Subtract2/2
  Data Type Conversion9/1 -> Delay/1
  Data Type Conversion10/1 -> Delay1/1
  Data Type Conversion11/1 -> Delay4/1
  Data Type Conversion12/1 -> Delay7/1
  Data Type Conversion13/1 -> Sum5/1, Delay8/1
  Data Type Conversion14/1 -> Delay9/1
  Gain/1 -> Data Type Conversion15/1
  Gain1/1 -> Out1/1
  Data Type Conversion15/1 -> Sum/1
  Data Type Conversion16/1 -> Gain1/1
  Sign/1 -> Data Type Conversion6/1
  Data Type Conversion3/1 -> Sign1/1, Subtract1/1
  Data Type Conversion5/1 -> Sign2/1, Subtract2/1
  Sign2/1 -> Data Type Conversion8/1

== system MIMO_FIXED/Transceiver7/ADC 1 ==
  In1 : Inport
  SigmaDelta ADC : Subsystem
  Switch : Switch  Criteria=u2 > Threshold  OutDataTypeStr=boolean
  Zero : Constant  Value=0
  bits 1&0 : Outport
  wires:
  SigmaDelta ADC/1(Out) -> Switch/1, Switch/2
  Zero/1 -> Switch/3
  In1/1 -> SigmaDelta ADC/1(In)
  Switch/1 -> bits 1&0/1

== system MIMO_FIXED/Transceiver7/CWM_RX2 ==
  In1 : Inport
  I_DDC : Inport  Port=2
  Q_DDC : Inport  Port=3
  Add : Sum
  Add1 : Sum  Inputs=-+
  Data Type Conversion{,1..9} (10 alike) : DataTypeConversion  OutDataTypeStr=fixdt(1,6,4)  SaturateOnIntegerOverflow=on
  Gain{,2,4,6} (4 alike) : Gain  Gain=-1
  Gain{1,3,5,7} (4 alike) : Gain
  Multiport Switch{,1,4..5} (4 alike) : MultiPortSwitch  DataPortOrder=Zero-based contiguous  Inputs=2  zeroidx=on  RndMeth=Nearest
  Trigonometric Function{,1,4..5} (4 alike) : Trigonometry
  Trigonometric Function{2..3,6..7} (4 alike) : Trigonometry  Operator=cos
  I` : Outport
  Q` : Outport  Port=2
  wires:
  Multiport Switch/1 -> Add1/1
  Add/1 -> Data Type Conversion8/1
  I_DDC/1 -> Multiport Switch1/1, Multiport Switch/1
  Gain2/1 -> Data Type Conversion6/1
  Trigonometric Function5/1 -> Gain5/1
  Data Type Conversion6/1 -> Multiport Switch1/2
  Data Type Conversion7/1 -> Multiport Switch/3
  Gain5/1 -> Data Type Conversion3/1
  Gain4/1 -> Data Type Conversion4/1
  Trigonometric Function1/1 -> Gain1/1
  Data Type Conversion2/1 -> Multiport Switch5/2
  Gain1/1 -> Data Type Conversion7/1
  Gain3/1 -> Data Type Conversion5/1
  Trigonometric Function3/1 -> Gain3/1
  Add1/1 -> Data Type Conversion9/1
  Gain/1 -> Data Type Conversion/1
  Trigonometric Function2/1 -> Gain2/1
  In1/1 -> Trigonometric Function3/1, Trigonometric Function6/1, Trigonometric Function7/1, Trigonometric Function5/1, Trigonometric Function4/1, Trigonometric Function2/1, Trigonometric Function1/1, Trigonometric Function/1
  Q_DDC/1 -> Multiport Switch5/1, Multiport Switch4/1
  Data Type Conversion1/1 -> Multiport Switch5/3
  Data Type Conversion4/1 -> Multiport Switch4/2
  Trigonometric Function6/1 -> Gain6/1
  Gain7/1 -> Data Type Conversion1/1
  Trigonometric Function4/1 -> Gain4/1
  Trigonometric Function/1 -> Gain/1
  Multiport Switch1/1 -> Add/1
  Multiport Switch4/1 -> Add/2
  Trigonometric Function7/1 -> Gain7/1
  Multiport Switch5/1 -> Add1/2
  Data Type Conversion3/1 -> Multiport Switch4/3
  Gain6/1 -> Data Type Conversion2/1
  Data Type Conversion/1 -> Multiport Switch/2
  Data Type Conversion5/1 -> Multiport Switch1/3
  Data Type Conversion8/1 -> I`/1
  Data Type Conversion9/1 -> Q`/1

== system MIMO_FIXED/Transceiver7/CWM_TX_Chain_1 ==
  PHI : Inport
  Processor_I : Inport  Port=2
  Processor_Q : Inport  Port=3
  Add : Sum  OutDataTypeStr=double  RndMeth=Round  SaturateOnIntegerOverflow=on
  Add1 : Sum  OutDataTypeStr=double
  Data Type Conversion : DataTypeConversion  OutDataTypeStr=fixdt(1,6,4)  SaturateOnIntegerOverflow=on
  Data Type Conversion1 : DataTypeConversion  OutDataTypeStr=fixdt(1,6,4)  RndMeth=Round  SaturateOnIntegerOverflow=on
  Data Type Conversion12 : DataTypeConversion  OutDataTypeStr=fixdt(1,16,9)  SaturateOnIntegerOverflow=on
  Data Type Conversion2 : DataTypeConversion  OutDataTypeStr=fixdt(1,6,4)  RndMeth=Round  SaturateOnIntegerOverflow=on
  Data Type Conversion3 : DataTypeConversion  OutDataTypeStr=fixdt(1,6,4)  SaturateOnIntegerOverflow=on
  Data Type Conversion4 : DataTypeConversion  OutDataTypeStr=fixdt(1,16,7)  SaturateOnIntegerOverflow=on
  Data Type Conversion5 : DataTypeConversion  OutDataTypeStr=fixdt(1,16,9)  SaturateOnIntegerOverflow=on
  Data Type Conversion6 : DataTypeConversion  OutDataTypeStr=fixdt(1,16,9)  SaturateOnIntegerOverflow=on
  Data Type Conversion7 : DataTypeConversion  OutDataTypeStr=fixdt(1,18,9)  SaturateOnIntegerOverflow=on
  Data Type Conversion8 : DataTypeConversion  OutDataTypeStr=fixdt(1,18,9)  SaturateOnIntegerOverflow=on
  Gain1 : Gain  Gain=-1
  Gain2 : Gain
  Gain3 : Gain
  Gain4 : Gain
  Product{,1..3} (4 alike) : Product
  Trigonometric Function1 : Trigonometry
  Trigonometric Function2 : Trigonometry  Operator=cos
  Trigonometric Function3 : Trigonometry  Operator=cos
  Trigonometric Function4 : Trigonometry
  I_1 : Outport
  Q_1 : Outport  Port=2
  wires:
  Trigonometric Function2/1 -> Gain2/1
  Gain2/1 -> Data Type Conversion/1
  Processor_Q/1 -> Product1/2, Product3/2
  Processor_I/1 -> Product2/1, Product/1
  Gain1/1 -> Data Type Conversion1/1
  Product/1 -> Data Type Conversion12/1
  Trigonometric Function1/1 -> Gain1/1
  PHI/1 -> Trigonometric Function2/1, Trigonometric Function1/1, Trigonometric Function4/1, Trigonometric Function3/1
  Data Type Conversion1/1 -> Product1/1
  Gain3/1 -> Data Type Conversion3/1
  Product2/1 -> Data Type Conversion5/1
  Data Type Conversion/1 -> Product/2
  Data Type Conversion2/1 -> Product2/2
  Data Type Conversion3/1 -> Product3/1
  Product3/1 -> Data Type Conversion6/1
  Trigonometric Function3/1 -> Gain3/1
  Product1/1 -> Data Type Conversion4/1
  Gain4/1 -> Data Type Conversion2/1
  Trigonometric Function4/1 -> Gain4/1
  Add1/1 -> Data Type Conversion8/1
  Data Type Conversion7/1 -> I_1/1
  Data Type Conversion8/1 -> Q_1/1
  Data Type Conversion12/1 -> Add/1
  Data Type Conversion4/1 -> Add/2
  Data Type Conversion5/1 -> Add1/1
  Data Type Conversion6/1 -> Add1/2
  Add/1 -> Data Type Conversion7/1

== system MIMO_FIXED/Transceiver7/DDC2 ==
  ODD_I : Inport
  EVEN_Q : Inport  Port=2
  Local_Oscilator1 : DiscretePulseGenerator  PhaseDelay=1  SampleTime=0.02
  Logical Operator : Logic  Operator=NXOR  AllPortsSameDT=off  OutDataTypeStr=boolean
  Logical Operator1 : Logic  Operator=NXOR  AllPortsSameDT=off  OutDataTypeStr=boolean
  NOT : Logic  Operator=NOT  IconShape=distinctive  AllPortsSameDT=off  OutDataTypeStr=boolean
  I_DDC : Outport
  Q_DDC : Outport  Port=2
  wires:
  Logical Operator/1 -> I_DDC/1
  EVEN_Q/1 -> Logical Operator1/2
  ODD_I/1 -> Logical Operator/1
  Logical Operator1/1 -> Q_DDC/1
  Local_Oscilator1/1 -> NOT/1
  NOT/1 -> Logical Operator1/1, Logical Operator/2

== system MIMO_FIXED/Transceiver7/DUC2 ==
  I_1 : Inport
  Q_1 : Inport  Port=2
  -cos : Sin  SineType=Sample based  Frequency=2*pi*100  Phase=pi/2  Samples=4  SampleTime=0.01  Offset=3
  -sin1 : Sin  SineType=Sample based  Frequency=(2*pi*100)/4  Samples=4  SampleTime=.01  Offset=2
  Add : Sum
  Constant : Constant  Value=0
  Constant1 : Constant  Value=0
  Data Type Conversion : DataTypeConversion  OutDataTypeStr=fixdt(1,2,0)  RndMeth=Round
  Data Type Conversion1 : DataTypeConversion  OutDataTypeStr=fixdt(1,2,0)  RndMeth=Round
  Data Type Conversion{2..3,5..6} (4 alike) : DataTypeConversion  OutDataTypeStr=fixdt(1,6,0)
  Data Type Conversion4 : DataTypeConversion  OutDataTypeStr=fixdt(1,7,0)
  Gain : Gain  Gain=-1
  Gain1 : Gain  Gain=-1
  Multiport Switch : MultiPortSwitch  DataPortOrder=Specify indices  DataPortIndices={1,0,-1}  RndMeth=Nearest
  Multiport Switch1 : MultiPortSwitch  DataPortOrder=Specify indices  DataPortIndices={1,0,-1}  RndMeth=Nearest
  Out2 : Outport
  wires:
  Constant/1 -> Multiport Switch1/3
  Q_1/1 -> Multiport Switch/2, Gain1/1
  I_1/1 -> Multiport Switch1/2, Gain/1
  Gain1/1 -> Data Type Conversion2/1
  -sin1/1 -> Data Type Conversion1/1
  -cos/1 -> Data Type Conversion/1
  Multiport Switch/1 -> Data Type Conversion5/1
  Add/1 -> Data Type Conversion4/1
  Multiport Switch1/1 -> Data Type Conversion6/1
  Constant1/1 -> Multiport Switch/3
  Gain/1 -> Data Type Conversion3/1
  Data Type Conversion/1 -> Multiport Switch1/1
  Data Type Conversion1/1 -> Multiport Switch/1
  Data Type Conversion2/1 -> Multiport Switch/4
  Data Type Conversion3/1 -> Multiport Switch1/4
  Data Type Conversion6/1 -> Add/1
  Data Type Conversion5/1 -> Add/2
  Data Type Conversion4/1 -> Out2/1

== system MIMO_FIXED/Transceiver7/Inter_Lever2 ==
  bits 1&0 : Inport
  Delay1 : Delay  DelayLength=1  InitialCondition=0
  Delay2 : Delay  DelayLength=1  InitialCondition=0
  Downsample : DownSample  RateOptions=Allow multirate processing
  Downsample1 : DownSample  RateOptions=Allow multirate processing
  ODD_I : Outport
  EVEN_Q : Outport  Port=2
  wires:
  Delay1/1 -> Downsample1/1
  Downsample/1 -> Delay2/1
  Downsample1/1 -> EVEN_Q/1
  bits 1&0/1 -> Delay1/1, Downsample/1
  Delay2/1 -> ODD_I/1

== system MIMO_FIXED/Transceiver7/Interpolation 1 ==
  Input : Inport
  Data Type Conversion2 : DataTypeConversion  OutDataTypeStr=fixdt(1,11,6)  SaturateOnIntegerOverflow=on
  Data Type Conversion5 : DataTypeConversion  OutDataTypeStr=fixdt(1,23,0)  SaturateOnIntegerOverflow=on
  Gain : Gain  Gain=512
  Gain1 : Gain  Gain=1/64
  Gain2 : Gain  Gain=1/512
  Gain3 : Gain  Gain=1/512
  Gain5 : Gain  Gain=64
  Half_band : Subsystem
  comb_filter : Subsystem
  Out1 : Outport
  wires:
  Input/1 -> Gain/1
  Gain5/1 -> comb_filter/1(In1)
  Gain1/1 -> Out1/1
  Data Type Conversion2/1 -> Gain5/1
  Gain2/1 -> Gain3/1
  Gain3/1 -> Data Type Conversion2/1
  Data Type Conversion5/1 -> Gain2/1
  Gain/1 -> Half_band/1(Input)
  Half_band/1(Out1) -> Data Type Conversion5/1
  comb_filter/1(Out1) -> Gain1/1

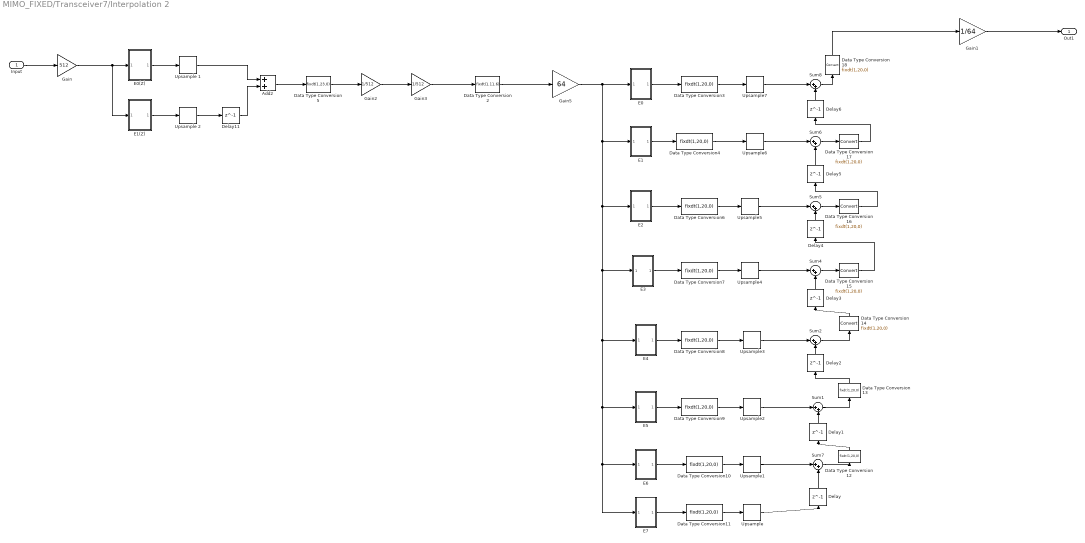
== system MIMO_FIXED/Transceiver7/Interpolation 2 ==
  Input : Inport
  Add2 : Sum
  Data Type Conversion{3..4,6..18} (15 alike) : DataTypeConversion  OutDataTypeStr=fixdt(1,20,0)  SaturateOnIntegerOverflow=on
  Data Type Conversion2 : DataTypeConversion  OutDataTypeStr=fixdt(1,11,6)  SaturateOnIntegerOverflow=on
  Data Type Conversion5 : DataTypeConversion  OutDataTypeStr=fixdt(1,23,0)  SaturateOnIntegerOverflow=on
  Delay{,1..6,11} (8 alike) : Delay  DelayLength=1
  E0 : Subsystem
  E0(Z) : Subsystem
  E1 : Subsystem
  E1(Z) : Subsystem
  E2 : Subsystem
  E3 : Subsystem
  E4 : Subsystem
  E5 : Subsystem
  E6 : Subsystem
  E7 : Subsystem
  Gain : Gain  Gain=512
  Gain1 : Gain  Gain=1/64
  Gain2 : Gain  Gain=1/512
  Gain3 : Gain  Gain=1/512
  Gain5 : Gain  Gain=64
  Sum{1..2,4..8} (7 alike) : Sum  Inputs=|++
  Upsample{,1..7} (8 alike) : dspsigops/Upsample  N=8  phase=0  RateOptions=Allow multirate processing  ic=0  mode=Unused parameter value
  Upsample 1 : dspsigops/Upsample  N=2  phase=0  RateOptions=Allow multirate processing  ic=0  mode=Unused parameter value
  Upsample 2 : dspsigops/Upsample  N=2  phase=0  RateOptions=Allow multirate processing  ic=0  mode=Unused parameter value
  Out1 : Outport
  wires:
  Upsample/1 -> Delay/1
  Delay5/1 -> Sum6/2
  Upsample6/1 -> Sum6/1
  Delay4/1 -> Sum5/2
  Delay3/1 -> Sum4/2
  Sum6/1 -> Data Type Conversion17/1
  Upsample1/1 -> Sum7/1
  Upsample2/1 -> Sum1/1
  Input/1 -> Gain/1
  Upsample 2/1 -> Delay11/1
  Delay6/1 -> Sum8/2
  E0/1(Out1) -> Data Type Conversion3/1
  Delay/1 -> Sum7/2
  E1/1(Out1) -> Data Type Conversion4/1
  Delay1/1 -> Sum1/2
  Sum5/1 -> Data Type Conversion16/1
  Sum4/1 -> Data Type Conversion15/1
  Upsample5/1 -> Sum5/1
  Upsample 1/1 -> Add2/1
  Upsample4/1 -> Sum4/1
  Delay11/1 -> Add2/2
  Sum2/1 -> Data Type Conversion14/1
  E3/1(Out1) -> Data Type Conversion7/1
  Delay2/1 -> Sum2/2
  Upsample7/1 -> Sum8/1
  Upsample3/1 -> Sum2/1
  E2/1(Out1) -> Data Type Conversion6/1
  E4/1(Out1) -> Data Type Conversion8/1
  E0(Z)/1(Out1) -> Upsample 1/1
  Data Type Conversion3/1 -> Upsample7/1
  Data Type Conversion4/1 -> Upsample6/1
  Data Type Conversion6/1 -> Upsample5/1
  Data Type Conversion7/1 -> Upsample4/1
  Data Type Conversion8/1 -> Upsample3/1
  Data Type Conversion9/1 -> Upsample2/1
  Data Type Conversion10/1 -> Upsample1/1
  Data Type Conversion11/1 -> Upsample/1
  Data Type Conversion12/1 -> Delay1/1
  Sum7/1 -> Data Type Conversion12/1
  Data Type Conversion13/1 -> Delay2/1
  Data Type Conversion14/1 -> Delay3/1
  Sum1/1 -> Data Type Conversion13/1
  Data Type Conversion15/1 -> Delay4/1
  Data Type Conversion16/1 -> Delay5/1
  Data Type Conversion17/1 -> Delay6/1
  Data Type Conversion18/1 -> Gain1/1
  Sum8/1 -> Data Type Conversion18/1
  E5/1(Out1) -> Data Type Conversion9/1
  E6/1(Out1) -> Data Type Conversion10/1
  E7/1(Out1) -> Data Type Conversion11/1
  Gain5/1 -> E0/1(In1), E7/1(In1), E6/1(In1), E5/1(In1), E4/1(In1), E3/1(In1), E2/1(In1), E1/1(In1)
  Gain1/1 -> Out1/1
  Gain/1 -> E0(Z)/1(Input), E1(Z)/1(Input1)
  Data Type Conversion2/1 -> Gain5/1
  Gain2/1 -> Gain3/1
  E1(Z)/1(Output) -> Upsample 2/1
  Gain3/1 -> Data Type Conversion2/1
  Add2/1 -> Data Type Conversion5/1
  Data Type Conversion5/1 -> Gain2/1

== system MIMO_FIXED/Transceiver7/Subsystem1 ==
  In1 : Inport
  Data Type Conversion : DataTypeConversion  OutDataTypeStr=fixdt(1,14,9)
  Data Type Conversion1 : DataTypeConversion  OutDataTypeStr=double
  Data Type Conversion{9..11,15} (4 alike) : DataTypeConversion  OutDataTypeStr=fixdt(1,13,9)
  Data Type Conversion12 : DataTypeConversion  OutDataTypeStr=fixdt(1,3,0)
  Data Type Conversion13 : DataTypeConversion  OutDataTypeStr=fixdt(1,3,0)
  Data Type Conversion14 : DataTypeConversion  OutDataTypeStr=fixdt(1,4,0)
  Data Type Conversion16 : DataTypeConversion  OutDataTypeStr=fixdt(1,4,0)
  Data Type Conversion2 : DataTypeConversion  OutDataTypeStr=fixdt(1,14,9)
  Data Type Conversion3 : DataTypeConversion  OutDataTypeStr=double
  Data Type Conversion4 : DataTypeConversion  OutDataTypeStr=fixdt(1,14,9)
  Data Type Conversion5 : DataTypeConversion  OutDataTypeStr=double
  Data Type Conversion6 : DataTypeConversion  OutDataTypeStr=fixdt(1,2,0)
  Data Type Conversion7 : DataTypeConversion  OutDataTypeStr=fixdt(1,2,0)
  Data Type Conversion8 : DataTypeConversion  OutDataTypeStr=fixdt(1,2,0)
  Delay{,1,4..9} (8 alike) : Delay  DelayLength=1
  Delay2 : Delay  DelayLength=5
  Delay3 : Delay  DelayLength=3
  Gain : Gain  Gain=1/16
  Gain1 : Gain  Gain=4
  Sign : Signum
  Sign1 : Signum
  Sign2 : Signum
  Subtract : Sum  Inputs=+-
  Subtract1 : Sum  Inputs=+-
  Subtract2 : Sum  Inputs=+-
  Sum{,1..2,4,6} (5 alike) : Sum  Inputs=|++
  Sum3 : Sum  Inputs=|+-
  Sum5 : Sum  Inputs=|+-
  Out1 : Outport
  wires:
  Sum/1 -> Data Type Conversion/1
  Sum2/1 -> Data Type Conversion4/1
  Delay4/1 -> Sum2/2
  Delay8/1 -> Sum5/2
  Sum4/1 -> Data Type Conversion13/1
  Subtract/1 -> Data Type Conversion9/1
  Delay5/1 -> Sum3/1, Delay6/1
  Sign1/1 -> Data Type Conversion7/1
  Delay1/1 -> Sum1/2, Sum2/1
  Sum1/1 -> Data Type Conversion2/1
  Subtract1/1 -> Data Type Conversion10/1
  Sum3/1 -> Data Type Conversion12/1
  Delay/1 -> Sum/2, Sum1/1
  Delay3/1 -> Sum4/1
  Delay7/1 -> Sum4/2
  Subtract2/1 -> Data Type Conversion11/1
  Delay6/1 -> Sum3/2
  Sum5/1 -> Data Type Conversion14/1
  Delay2/1 -> Sum6/1
  Delay9/1 -> Sum6/2
  In1/1 -> Gain/1
  Sum6/1 -> Data Type Conversion16/1
  Data Type Conversion/1 -> Data Type Conversion1/1
  Data Type Conversion1/1 -> Subtract/1, Sign/1
  Data Type Conversion2/1 -> Data Type Conversion3/1
  Data Type Conversion4/1 -> Data Type Conversion5/1
  Data Type Conversion6/1 -> Subtract/2, Delay2/1
  Data Type Conversion7/1 -> Subtract1/2, Delay3/1
  Data Type Conversion8/1 -> Delay5/1, Subtract2/2
  Data Type Conversion9/1 -> Delay/1
  Data Type Conversion10/1 -> Delay1/1
  Data Type Conversion11/1 -> Delay4/1
  Data Type Conversion12/1 -> Delay7/1
  Data Type Conversion13/1 -> Sum5/1, Delay8/1
  Data Type Conversion14/1 -> Delay9/1
  Gain/1 -> Data Type Conversion15/1
  Gain1/1 -> Out1/1
  Data Type Conversion15/1 -> Sum/1
  Data Type Conversion16/1 -> Gain1/1
  Sign/1 -> Data Type Conversion6/1
  Data Type Conversion3/1 -> Sign1/1, Subtract1/1
  Data Type Conversion5/1 -> Sign2/1, Subtract2/1
  Sign2/1 -> Data Type Conversion8/1

== system MIMO_FIXED/Transceiver7/Subsystem2 ==
  In1 : Inport
  Data Type Conversion : DataTypeConversion  OutDataTypeStr=fixdt(1,14,9)
  Data Type Conversion1 : DataTypeConversion  OutDataTypeStr=double
  Data Type Conversion{9..11,15} (4 alike) : DataTypeConversion  OutDataTypeStr=fixdt(1,13,9)
  Data Type Conversion12 : DataTypeConversion  OutDataTypeStr=fixdt(1,3,0)
  Data Type Conversion13 : DataTypeConversion  OutDataTypeStr=fixdt(1,3,0)
  Data Type Conversion14 : DataTypeConversion  OutDataTypeStr=fixdt(1,4,0)
  Data Type Conversion16 : DataTypeConversion  OutDataTypeStr=fixdt(1,4,0)
  Data Type Conversion2 : DataTypeConversion  OutDataTypeStr=fixdt(1,14,9)
  Data Type Conversion3 : DataTypeConversion  OutDataTypeStr=double
  Data Type Conversion4 : DataTypeConversion  OutDataTypeStr=fixdt(1,14,9)
  Data Type Conversion5 : DataTypeConversion  OutDataTypeStr=double
  Data Type Conversion6 : DataTypeConversion  OutDataTypeStr=fixdt(1,2,0)
  Data Type Conversion7 : DataTypeConversion  OutDataTypeStr=fixdt(1,2,0)
  Data Type Conversion8 : DataTypeConversion  OutDataTypeStr=fixdt(1,2,0)
  Delay{,1,4..9} (8 alike) : Delay  DelayLength=1
  Delay2 : Delay  DelayLength=5
  Delay3 : Delay  DelayLength=3
  Gain : Gain  Gain=1/16
  Gain1 : Gain  Gain=4
  Sign : Signum
  Sign1 : Signum
  Sign2 : Signum
  Subtract : Sum  Inputs=+-
  Subtract1 : Sum  Inputs=+-
  Subtract2 : Sum  Inputs=+-
  Sum{,1..2,4,6} (5 alike) : Sum  Inputs=|++
  Sum3 : Sum  Inputs=|+-
  Sum5 : Sum  Inputs=|+-
  Out1 : Outport
  wires:
  Sum/1 -> Data Type Conversion/1
  Sum2/1 -> Data Type Conversion4/1
  Delay4/1 -> Sum2/2
  Delay8/1 -> Sum5/2
  Sum4/1 -> Data Type Conversion13/1
  Subtract/1 -> Data Type Conversion9/1
  Delay5/1 -> Sum3/1, Delay6/1
  Sign1/1 -> Data Type Conversion7/1
  Delay1/1 -> Sum1/2, Sum2/1
  Sum1/1 -> Data Type Conversion2/1
  Subtract1/1 -> Data Type Conversion10/1
  Sum3/1 -> Data Type Conversion12/1
  Delay/1 -> Sum/2, Sum1/1
  Delay3/1 -> Sum4/1
  Delay7/1 -> Sum4/2
  Subtract2/1 -> Data Type Conversion11/1
  Delay6/1 -> Sum3/2
  Sum5/1 -> Data Type Conversion14/1
  Delay2/1 -> Sum6/1
  Delay9/1 -> Sum6/2
  In1/1 -> Gain/1
  Sum6/1 -> Data Type Conversion16/1
  Data Type Conversion/1 -> Data Type Conversion1/1
  Data Type Conversion1/1 -> Subtract/1, Sign/1
  Data Type Conversion2/1 -> Data Type Conversion3/1
  Data Type Conversion4/1 -> Data Type Conversion5/1
  Data Type Conversion6/1 -> Subtract/2, Delay2/1
  Data Type Conversion7/1 -> Subtract1/2, Delay3/1
  Data Type Conversion8/1 -> Delay5/1, Subtract2/2
  Data Type Conversion9/1 -> Delay/1
  Data Type Conversion10/1 -> Delay1/1
  Data Type Conversion11/1 -> Delay4/1
  Data Type Conversion12/1 -> Delay7/1
  Data Type Conversion13/1 -> Sum5/1, Delay8/1
  Data Type Conversion14/1 -> Delay9/1
  Gain/1 -> Data Type Conversion15/1
  Gain1/1 -> Out1/1
  Data Type Conversion15/1 -> Sum/1
  Data Type Conversion16/1 -> Gain1/1
  Sign/1 -> Data Type Conversion6/1
  Data Type Conversion3/1 -> Sign1/1, Subtract1/1
  Data Type Conversion5/1 -> Sign2/1, Subtract2/1
  Sign2/1 -> Data Type Conversion8/1

== system MIMO_FIXED/decimation1/E0(Z) ==
  Input : Inport
  Data Type Conversion5 : DataTypeConversion  OutDataTypeStr=fixdt(1,18,0)  SaturateOnIntegerOverflow=on
  Delay : Delay  DelayLength=5
  Gain : Gain  Gain=256
  Out1 : Outport
  wires:
  Input/1 -> Gain/1
  Delay/1 -> Out1/1
  Data Type Conversion5/1 -> Delay/1
  Gain/1 -> Data Type Conversion5/1

== system MIMO_FIXED/decimation1/E1(Z) ==
  Input1 : Inport
  10-12 : Gain  Gain=158
  2-20 : Gain
  4-18 : Gain  Gain=-4
  6-16 : Gain  Gain=13
  8-14 : Gain  Gain=-40
  Add{7..10,12..16} (9 alike) : Sum
  Data Type Conversion1 : DataTypeConversion  OutDataTypeStr=fixdt(1,10,0)  SaturateOnIntegerOverflow=on
  Data Type Conversion{5,10..14} (6 alike) : DataTypeConversion  OutDataTypeStr=fixdt(1,18,0)  SaturateOnIntegerOverflow=on
  Data Type Conversion2 : DataTypeConversion  OutDataTypeStr=fixdt(1,12,0)  SaturateOnIntegerOverflow=on
  Data Type Conversion3 : DataTypeConversion  OutDataTypeStr=fixdt(1,14,0)  SaturateOnIntegerOverflow=on
  Data Type Conversion4 : DataTypeConversion  OutDataTypeStr=fixdt(1,16,0)  SaturateOnIntegerOverflow=on
  Data Type Conversion6 : DataTypeConversion  OutDataTypeStr=fixdt(1,12,0)  SaturateOnIntegerOverflow=on
  Data Type Conversion7 : DataTypeConversion  OutDataTypeStr=fixdt(1,14,0)  SaturateOnIntegerOverflow=on
  Data Type Conversion8 : DataTypeConversion  OutDataTypeStr=fixdt(1,15,0)  SaturateOnIntegerOverflow=on
  Data Type Conversion9 : DataTypeConversion  OutDataTypeStr=fixdt(1,17,0)  SaturateOnIntegerOverflow=on
  Delay{21,23,25,27,29,31,33,35,37} (9 alike) : Delay  DelayLength=1
  Output : Outport
  wires:
  8-14/1 -> Data Type Conversion4/1
  Delay29/1 -> Add12/2  "x[n-11]"
  Add14/1 -> Data Type Conversion12/1
  Input1/1 -> 2-20/1, 10-12/1, 8-14/1, 6-16/1, 4-18/1
  Delay33/1 -> Add14/2
  Add12/1 -> Data Type Conversion10/1
  10-12/1 -> Data Type Conversion5/1
  Delay37/1 -> Add16/2  "x[n-19]"
  6-16/1 -> Data Type Conversion3/1
  Delay25/1 -> Add9/2  "x[n-7]"
  Add15/1 -> Data Type Conversion13/1
  Delay23/1 -> Add8/2  "x[n-5]"
  Delay27/1 -> Add10/2  "x[n-9]"
  Delay31/1 -> Add13/2  "x[n-13]"
  Delay35/1 -> Add15/2  "x[n-17]"
  Delay21/1 -> Add7/2  "x[n-3]"
  Add13/1 -> Data Type Conversion11/1
  Add10/1 -> Data Type Conversion9/1
  Data Type Conversion1/1 -> Delay21/1, Add16/1
  Data Type Conversion2/1 -> Add7/1, Add15/1
  Data Type Conversion3/1 -> Add8/1, Add14/1
  Data Type Conversion4/1 -> Add9/1, Add13/1
  Data Type Conversion5/1 -> Add10/1, Add12/1
  Data Type Conversion6/1 -> Delay23/1
  Add8/1 -> Data Type Conversion7/1
  Data Type Conversion7/1 -> Delay25/1
  Data Type Conversion8/1 -> Delay27/1
  Data Type Conversion9/1 -> Delay29/1
  Data Type Conversion10/1 -> Delay31/1
  Data Type Conversion11/1 -> Delay33/1
  Data Type Conversion12/1 -> Delay35/1
  Data Type Conversion13/1 -> Delay37/1
  Data Type Conversion14/1 -> Output/1
  2-20/1 -> Data Type Conversion1/1
  4-18/1 -> Data Type Conversion2/1
  Add7/1 -> Data Type Conversion6/1
  Add16/1 -> Data Type Conversion14/1
  Add9/1 -> Data Type Conversion8/1
